simulink library "tqd"  (R2021b)
settings: Solver=VariableStepAuto  StartTime=0.0  StopTime=10.0  RelTol=1e-3
undefined symbols (not defined in the file or in its folder): ATQD_APSDecReq_X_kph, ATQD_APSDecReq_Y_mps2, ATQD_APSDecReqCMD_X_kph, ATQD_APSDecReqTs_X_pct, ATQD_APSDecTimeGain_X_Deg, ATQD_APSDecTimeGain_Y_s, ATQD_APSReqLowSpd_X_Deg, ATQD_AutoHoldReleaseBPS_X_Deg, ATQD_AWDLoadTrqnsGain_X_kg, ATQD_AWDLoadTrqnsGain_Y_pct, ATQD_BOSEnBPSPosn_X_kph, ATQD_BOSMap_X_rpm, ATQD_BOSMap_Y_pct, ATQD_CreepBaseTqD_X_kph, ATQD_CreepBaseTqD_Y_Deg, ATQD_CreepBaseTqR_X_kph, ATQD_CreepBaseTqR_Y_Deg, ATQD_CreepBPSDisPosn_X_Deg, ATQD_CreepBPSDisPosnR_X_Deg, ATQD_CreepBPSEnPosn_X_Deg, ATQD_CreepBPSEnPosnR_X_Deg, ATQD_CreepDeltaTq_X_kph, ATQD_CreepIterm_X_kph, ATQD_CreepIterm_Y_kph, ATQD_CreepItermMaxLimit_X_pct, ATQD_CreepPreloadTime_X_kph, ATQD_CreepPreloadTq_X_kph, ATQD_CreepPreloadTq_Y_s, ATQD_CreepProtTq_X_Deg, ATQD_CreepPterm_X_kph, ATQD_CreepPterm_Y_kph, ATQD_ECOTqMapD_X_rpm, ATQD_ECOTqMapD_Y_pct, ATQD_EOPDTqMapDCon_X_rpm, ATQD_EOPDTqMapDCon_Y_Deg, ATQD_EstInitVehWeight_X_c, ATQD_LHMRollGenMapD_X_rpm, ATQD_LHMRollGenMapD_Y_rpm, ATQD_LHMTqMapD_X_rpm, ATQD_LHMTqMapD_Y_pct, ATQD_NL1TqMapD_X_rpm, ATQD_NL1TqMapD_Y_pct, ATQD_NOPDTqMapDCon_X_rpm, ATQD_NOPDTqMapDCon_Y_Deg, ATQD_NRMRrEDUSpRat_X_rpm, ATQD_NRMRrEDUSpRat_Y_Nm, ATQD_OPDHoldDownRelDelay_X_Deg, ATQD_OPDHoldEnSpd_X_Deg, ATQD_OPDHoldRelDetTime_X_Deg, ATQD_OPDHoldReleaseTq_X_Deg, ATQD_OrigPedTqLowLim_X_Deg, ATQD_OrigPedTqLowLim_Y_pct, ATQD_PedalMapClimbUpLim_X_rpm, ATQD_PedalMapClimbUpLim_Y_Deg, ATQD_PreLoadTq_X_s, ATQD_RollGenMapEL1_X_rpm, ATQD_RollGenMapEL1_Y_rpm, ATQD_SL1TqMapD_X_rpm, ATQD_SL1TqMapD_Y_pct, ATQD_SlideRegenTqGain_X_Gps ... (+487)
libraries: hcu_lib x83, simulink x73, tqr x1
(part 14 of 19)

== system tqd/TQD/TorqueDemand/TorqueModule/AvaliableTqLimit/TorqueCapacityCalcalation/CapacityDistribution ==
  VTQD_FrEDUSpRat_cmd : Inport
  VTQD_RrEDUSpRat_rat : Inport  Port=2
  VTQD_TMPwrAvailDchrg_kW : Inport  Port=3
  VINP_HVBPwrAvailChrg_kw : Inport  Port=4
  Abs1 : Abs
  Product{,1,4..5} (4 alike) : Product
  VTQD_FrHVBPwrAvailDchrg_kw : Outport
  VTQD_RrHVBPwrAvailDchrg_kw : Outport  Port=2
  VTQD_FrHVBPwrAvailChrg_kw : Outport  Port=3
  VTQD_RrHVBPwrAvailChrg_kw : Outport  Port=4
  wires:
  VTQD_RrEDUSpRat_rat/1 -> [VTQD_RrEDUSpRat_rat]
  VTQD_FrEDUSpRat_cmd/1 -> [VTQD_FrEDUSpRat_rat]
  VINP_HVBPwrAvailChrg_kw/1 -> Abs1/1
  Product4/1 -> VTQD_FrHVBPwrAvailChrg_kw/1
  Product5/1 -> VTQD_RrHVBPwrAvailChrg_kw/1
  Product1/1 -> VTQD_RrHVBPwrAvailDchrg_kw/1  "VTQD_RrHVBPwrAvailDchrg_kW"
  [VTQD_FrEDUSpRat_rat] -> Product4/1
  [VTQD_FrEDUSpRat_rat] -> Product/1
  Abs1/1 -> Product4/2, Product5/1
  VTQD_TMPwrAvailDchrg_kW/1 -> Product1/1, Product/2
  [VTQD_RrEDUSpRat_rat] -> Product5/2
  Product/1 -> VTQD_FrHVBPwrAvailDchrg_kw/1  "VTQD_FrHVBPwrAvailDchrg_kW"
  [VTQD_RrEDUSpRat_rat] -> Product1/2

== system tqd/TQD/TorqueDemand/TorqueModule/AvaliableTqLimit/TorqueCapacityCalcalation/Generation ==
  VTQD_FrShaftSpd_rpm : Inport
  VTQD_RrShaftSpd_rpm : Inport  Port=2
  VTQD_FrHVBPwrAvailChrg_kw : Inport  Port=3
  VTQD_RrHVBPwrAvailChrg_kw : Inport  Port=4
  KTQD_FrBatapCont_factor : Inport  Port=5
  KTQD_RrBatapCont_factor : Inport  Port=6
  VINP_FrRegenAvailTq_Nm : Inport  Port=7
  VINP_RrRegenAvailTq_Nm : Inport  Port=8
  VTQD_GearActualPosn_enum : Inport  Port=9
  VINP_VehicleType_enum : Inport  Port=10
  Abs2 : Abs
  Abs6 : Abs
  Constant : Constant  Value=KTQD_WhlTqCapGenFr_Nm_ovrdflg
  Constant1 : Constant  Value=KTQD_WhlTqCapGenFr_Nm_ovrdval
  Constant10 : Constant  Value=ENUM_GEARACTUALPOSN_P  OutDataTypeStr=single
  Constant11 : Constant  Value=ENUM_GEARACTUALPOSN_P  OutDataTypeStr=single
  Constant12 : Constant  Value=ENUM_VEHICLETYPE_D31L24
  Constant13 : Constant  Value=ZERO_FLOAT
  Constant14 : Constant  Value=ENUM_GEARACTUALPOSN_N  OutDataTypeStr=single
  Constant19 : Constant  Value=ENUM_VEHICLETYPE_D31L24
  Constant2 : Constant  Value=KTQD_RrTMSpdMin_rpm  OutDataTypeStr=single
  Constant3 : Constant  Value=KTQD_WhlTqCapGenRr_Nm_ovrdflg
  Constant4 : Constant  Value=KTQD_RrTMTotalGearRatio_gain  OutDataTypeStr=single
  Constant5 : Constant  Value=KTQD_FrTMSpdMin_rpm  OutDataTypeStr=single
  Constant6 : Constant  Value=KTQD_FrTMTotalGearRatio_gain  OutDataTypeStr=single
  Constant7 : Constant  Value=KTQD_WhlTqCapGenRr_Nm_ovrdval
  Constant8 : Constant  Value=ZERO_FLOAT
  Constant9 : Constant  Value=ENUM_GEARACTUALPOSN_N  OutDataTypeStr=single
  Equal{1..4} (4 alike) : RelationalOperator  Operator===  OutDataTypeStr=boolean  RndMeth=Simplest
  Equal5 : RelationalOperator  Operator=~=  OutDataTypeStr=boolean  RndMeth=Simplest
  Equal6 : RelationalOperator  Operator=~=  OutDataTypeStr=boolean  RndMeth=Simplest
  Fcn : Fcn  Expr=u[1]/u[2]/pi*u[3]
  Fcn2 : Fcn  Expr=u[1]/u[2]/pi*u[3]
  Gain1 : Gain  Gain=-1
  Gain4 : Gain  Gain=-1
  Logical Operator1 : Logic  AllPortsSameDT=off  OutDataTypeStr=boolean
  Logical Operator2 : Logic  AllPortsSameDT=off  OutDataTypeStr=boolean
  Max{,1..2,4} (4 alike) : MinMax  Function=max  Inputs=2
  Mux : Mux  Inputs=3
  Mux2 : Mux  Inputs=3
  OR1 : Logic  Operator=OR  AllPortsSameDT=off  OutDataTypeStr=boolean
  OR2 : Logic  Operator=OR  AllPortsSameDT=off  OutDataTypeStr=boolean
  Product1 : Product
  Product2 : Product
  Saturation1 : Saturate  UpperLimit=0  LowerLimit=KTQD_FrLowTheldTrq_Nm
      settings: AttributesFormatString=|
      | Upper Limit :%<UpperLimit>
      | Lower Limit :%<LowerLimit>
  Saturation2 : Saturate  UpperLimit=0  LowerLimit=KTQD_RrLowTheldTrq_Nm
      settings: AttributesFormatString=|
      | Upper Limit :%<UpperLimit>
      | Lower Limit :%<LowerLimit>
  Switch : Switch  Criteria=u2 ~= 0
      settings: AttributesFormatString=<%<Criteria>>
  Switch1 : Switch  Criteria=u2 ~= 0
      settings: AttributesFormatString=<%<Criteria>>
  Switch2 : Switch  Criteria=u2 > Threshold
  Switch3 : Switch  Criteria=u2 > Threshold
  VTQD_WhlTqCapGenFr_Nm : Outport
  VTQD_WhlTqCapGenRr_Nm : Outport  Port=2
  wires:
  Gain1/1 -> Saturation2/1
  Gain4/1 -> Saturation1/1
  Switch1/1 -> VTQD_WhlTqCapGenRr_Nm/1  "VTQD_WhlTqCapGenRr_Nm"
  Constant3/1 -> Switch1/2
  Constant7/1 -> Switch1/1
  Switch/1 -> VTQD_WhlTqCapGenFr_Nm/1  "VTQD_WhlTqCapGenFr_Nm"
  Constant1/1 -> Switch/1
  Constant/1 -> Switch/2
  VTQD_RrHVBPwrAvailChrg_kw/1 -> [VTQD_RrHVBPwrAvailChrg_kw]
  KTQD_FrBatapCont_factor/1 -> [KTQD_FrBatapCont_factor]
  VTQD_FrHVBPwrAvailChrg_kw/1 -> [VTQD_FrHVBPwrAvailChrg_kw]
  VTQD_FrShaftSpd_rpm/1 -> [VTQD_FrShaftSpd_rpm]
  VTQD_RrShaftSpd_rpm/1 -> [VTQD_RrShaftSpd_rpm]
  KTQD_RrBatapCont_factor/1 -> [KTQD_RrBatapCont_factor]
  Fcn2/1 -> Gain1/1
  Max1/1 -> Mux2/2
  Abs2/1 -> Max1/1
  Mux2/1 -> Fcn2/1
  Constant2/1 -> Max1/2
  [KTQD_RrBatapCont_factor] -> Mux2/3
  [VTQD_RrShaftSpd_rpm] -> Abs2/1
  [VTQD_RrHVBPwrAvailChrg_kw] -> Mux2/1
  Fcn/1 -> Gain4/1
  Abs6/1 -> Max4/1
  [VTQD_FrHVBPwrAvailChrg_kw] -> Mux/1
  Constant5/1 -> Max4/2
  [VTQD_FrShaftSpd_rpm] -> Abs6/1
  [KTQD_FrBatapCont_factor] -> Mux/3
  Mux/1 -> Fcn/1
  Max4/1 -> Mux/2
  Saturation1/1 -> Max2/1
  Max2/1 -> Switch/3
  Saturation2/1 -> Max/1
  Max/1 -> Switch1/3
  VINP_RrRegenAvailTq_Nm/1 -> [VINP_RrRegenAvailTq_Nm]
  VINP_FrRegenAvailTq_Nm/1 -> [VINP_FrRegenAvailTq_Nm]
  VTQD_GearActualPosn_enum/1 -> [VTQD_GearActualPosn_enum]
  [VINP_FrRegenAvailTq_Nm] -> Product2/1
  Equal2/1 -> OR2/2
  Equal4/1 -> OR2/1
  Constant10/1 -> Equal4/2
  Constant6/1 -> Product2/2
  Constant9/1 -> Equal2/2
  [VTQD_GearActualPosn_enum] -> Equal2/1
  Constant8/1 -> Switch2/1
  Product2/1 -> Switch2/3
  [VTQD_GearActualPosn_enum] -> Equal4/1
  Switch2/1 -> Max2/2
  Constant4/1 -> Product1/2
  [VINP_RrRegenAvailTq_Nm] -> Product1/1
  Switch3/1 -> Max/2
  [VINP_VehicleType_enum] -> Equal6/1
  Equal6/1 -> Logical Operator1/2
  Constant19/1 -> Equal6/2
  OR2/1 -> Logical Operator1/1
  Logical Operator1/1 -> Switch2/2
  OR1/1 -> Logical Operator2/1
  Equal5/1 -> Logical Operator2/2
  Constant12/1 -> Equal5/2
  [VINP_VehicleType_enum] -> Equal5/1
  Constant14/1 -> Equal1/2
  Equal1/1 -> OR1/2
  Constant13/1 -> Switch3/1
  [VTQD_GearActualPosn_enum] -> Equal1/1
  Constant11/1 -> Equal3/2
  [VTQD_GearActualPosn_enum] -> Equal3/1
  Logical Operator2/1 -> Switch3/2
  Equal3/1 -> OR1/1
  Product1/1 -> Switch3/3
  VINP_VehicleType_enum/1 -> [VINP_VehicleType_enum]

== system tqd/TQD/TorqueDemand/TorqueModule/AvaliableTqLimit/TorqueCapacityCalcalation/Motoring ==
  VTQD_FrShaftSpd_rpm : Inport
  VTQD_RrShaftSpd_rpm : Inport  Port=2
  VTQD_FrHVBPwrAvailDchrg_kw : Inport  Port=3
  VTQD_RrHVBPwrAvailDchrg_kw : Inport  Port=4
  KTQD_FrBatapCont_factor : Inport  Port=5
  KTQD_RrBatapCont_factor : Inport  Port=6
  VINP_HVBCellVoltMax_mV : Inport  Port=7
  VINP_HVBCellVoltMin_mV : Inport  Port=8
  VINP_HVBSOH_pct : Inport  Port=9
  VINP_FrMotorAvailTq_Nm : Inport  Port=10
  VINP_RrMotorAvailTq_Nm : Inport  Port=11
  VTQD_GearActualPosn_enum : Inport  Port=12
  VINP_VehicleType_enum : Inport  Port=13
  Abs : Abs
  Abs2 : Abs
  Add : Sum  Commented=on  Inputs=+-
  Constant : Constant  Value=KTQD_WhlTqCapMotFr_Nm_ovrdflg
  Constant1 : Constant  Value=KTQD_FrTMSpdMin_rpm  OutDataTypeStr=single
  Constant10 : Constant  Value=KTQD_FrTMTotalGearRatio_gain  OutDataTypeStr=single
  Constant11 : Constant  Value=KTQD_RrTMTotalGearRatio_gain  OutDataTypeStr=single
  Constant{2,4,12..13} (4 alike) : Constant  Value=ZERO_FLOAT
  Constant14 : Constant  Value=ENUM_GEARACTUALPOSN_N  OutDataTypeStr=single
  Constant15 : Constant  Value=ENUM_GEARACTUALPOSN_P  OutDataTypeStr=single
  Constant16 : Constant  Value=ENUM_GEARACTUALPOSN_N  OutDataTypeStr=single
  Constant17 : Constant  Value=ENUM_GEARACTUALPOSN_P  OutDataTypeStr=single
  Constant18 : Constant  Value=ENUM_VEHICLETYPE_D31L24
  Constant19 : Constant  Value=ENUM_VEHICLETYPE_D31L24
  Constant3 : Constant  Value=KTQD_RrTMSpdMin_rpm  OutDataTypeStr=single
  Constant5 : Constant  Value=KTQD_WhlTqCapMotFr_Nm_ovrdval
  Constant6 : Constant  Value=KTQD_WhlTqCapMotRr_Nm_ovrdflg
  Constant7 : Constant  Value=KTQD_WhlTqCapMotRr_Nm_ovrdval
  Constant8 : Constant  Value=KTQD_FrUppTheldTrq_Nm
  Constant9 : Constant  Value=KTQD_RrUppTheldTrq_Nm
  Equal{1..3,5} (4 alike) : RelationalOperator  Operator===  OutDataTypeStr=boolean  RndMeth=Simplest
  Equal4 : RelationalOperator  Operator=~=  OutDataTypeStr=boolean  RndMeth=Simplest
  Equal6 : RelationalOperator  Operator=~=  OutDataTypeStr=boolean  RndMeth=Simplest
  Fcn : Fcn  Expr=u[1]/u[2]/pi*u[3]
  Fcn2 : Fcn  Expr=u[1]/u[2]/pi*u[3]
  From3 : From  Commented=on  GotoTag=VINP_HVBCellVoltMax_mV
  From4 : From  Commented=on  GotoTag=VINP_HVBCellVoltMin_mV
  From5 : From  Commented=on  GotoTag=VTQD_HCBCellVoltDev_mV
  From6 : From  Commented=on  GotoTag=VINP_HVBSOH_pct
  Goto7 : Goto  Commented=on  GotoTag=VTQD_HCBCellVoltDev_mV
  Goto9 : Goto  Commented=on  GotoTag=VTQD_WhlTqCapMotGain_c
  Logical Operator : Logic  AllPortsSameDT=off  OutDataTypeStr=boolean
  Logical Operator1 : Logic  AllPortsSameDT=off  OutDataTypeStr=boolean
  MTQD_WhlTqCapMotGain_Z_c : Lookup_n-D  Commented=on  BreakpointsForDimension1=ATQD_WhlTqCapMotGain_Y_mV  BreakpointsForDimension2=ATQD_WhlTqCapMotGain_X_pct  Table=MTQD_WhlTqCapMotGain_Z_c  InternalRulePriority=Speed  RndMeth=Simplest  InputSameDT=on
      settings: InputPortMap=u0,u1
  Max{,1..3} (4 alike) : MinMax  Function=max  Inputs=2
  Min : MinMax  Inputs=3
  Min1 : MinMax  Inputs=3
  Mux : Mux  Inputs=3
  Mux2 : Mux  Inputs=3
  OR1 : Logic  Operator=OR  AllPortsSameDT=off  OutDataTypeStr=boolean
  OR2 : Logic  Operator=OR  AllPortsSameDT=off  OutDataTypeStr=boolean
  Product : Product
  Product1 : Product
  Switch : Switch  Criteria=u2 ~= 0
      settings: AttributesFormatString=<%<Criteria>>
  Switch1 : Switch  Criteria=u2 ~= 0
      settings: AttributesFormatString=<%<Criteria>>
  Switch2 : Switch  Criteria=u2 > Threshold
  Switch3 : Switch  Criteria=u2 > Threshold
  VTQD_WhlTqCapMotFr_Nm : Outport
  VTQD_WhlTqCapMotRr_Nm : Outport  Port=2
  wires:
  Fcn2/1 -> Min1/1
  Switch1/1 -> VTQD_WhlTqCapMotRr_Nm/1  "VTQD_WhlTqCapMotRr_Nm"
  Constant7/1 -> Switch1/1
  Constant6/1 -> Switch1/2
  Constant5/1 -> Switch/1
  Constant/1 -> Switch/2
  Switch/1 -> VTQD_WhlTqCapMotFr_Nm/1  "VTQD_WhlTqCapMotFr_Nm"
  VTQD_RrHVBPwrAvailDchrg_kw/1 -> [VTQD_RrHVBPwrAvailDchrg_kw]
  KTQD_RrBatapCont_factor/1 -> [KTQD_RrBatapCont_factor]
  VTQD_RrShaftSpd_rpm/1 -> [VTQD_RrShaftSpd_rpm]
  Abs2/1 -> Max2/1
  [VTQD_RrHVBPwrAvailDchrg_kw] -> Mux2/1
  Constant3/1 -> Max2/2
  [VTQD_RrShaftSpd_rpm] -> Abs2/1
  Mux2/1 -> Fcn2/1
  Max2/1 -> Mux2/2
  [VTQD_FrHVBPwrAvailDchrg_kw] -> Mux/1
  Max/1 -> Mux/2
  [VTQD_FrShaftSpd_rpm] -> Abs/1
  KTQD_FrBatapCont_factor/1 -> [KTQD_FrBatapCont_factor]
  VTQD_FrHVBPwrAvailDchrg_kw/1 -> [VTQD_FrHVBPwrAvailDchrg_kw]
  Abs/1 -> Max/1
  Fcn/1 -> Min/1
  Mux/1 -> Fcn/1
  VTQD_FrShaftSpd_rpm/1 -> [VTQD_FrShaftSpd_rpm]
  Constant1/1 -> Max/2
  Constant8/1 -> Min/2
  Min/1 -> Max1/1
  Constant2/1 -> Max1/2
  Constant9/1 -> Min1/2
  Constant4/1 -> Max3/2
  VINP_HVBCellVoltMin_mV/1 -> [VINP_HVBCellVoltMin_mV]
  VINP_HVBSOH_pct/1 -> [VINP_HVBSOH_pct]
  VINP_HVBCellVoltMax_mV/1 -> [VINP_HVBCellVoltMax_mV]
  Add/1 -> Goto7/1  "VTQD_HCBCellVoltDev_mV"
  From3/1 -> Add/1
  From4/1 -> Add/2
  From5/1 -> MTQD_WhlTqCapMotGain_Z_c/1
  [KTQD_FrBatapCont_factor] -> Mux/3
  [KTQD_RrBatapCont_factor] -> Mux2/3
  MTQD_WhlTqCapMotGain_Z_c/1 -> Goto9/1  "VTQD_WhlTqCapMotGain_c"
  Max1/1 -> Switch/3
  Max3/1 -> Switch1/3
  From6/1 -> MTQD_WhlTqCapMotGain_Z_c/2
  VINP_FrMotorAvailTq_Nm/1 -> [VINP_FrMotorAvailTq_Nm]
  VINP_RrMotorAvailTq_Nm/1 -> [VINP_RrMotorAvailTq_Nm]
  Min1/1 -> Max3/1
  Constant10/1 -> Product/2
  [VINP_FrMotorAvailTq_Nm] -> Product/1
  Constant16/1 -> Equal1/2
  Constant11/1 -> Product1/2
  Switch3/1 -> Min1/3
  [VINP_RrMotorAvailTq_Nm] -> Product1/1
  Equal3/1 -> OR1/1
  [VTQD_GearActualPosn_enum] -> Equal3/1
  Product1/1 -> Switch3/3
  Constant13/1 -> Switch3/1
  [VTQD_GearActualPosn_enum] -> Equal1/1
  Equal1/1 -> OR1/2
  Constant17/1 -> Equal3/2
  VTQD_GearActualPosn_enum/1 -> [VTQD_GearActualPosn_enum]
  [VINP_VehicleType_enum] -> Equal4/1
  Equal4/1 -> Logical Operator/2
  Constant18/1 -> Equal4/2
  OR1/1 -> Logical Operator/1
  Logical Operator/1 -> Switch3/2
  Equal6/1 -> Logical Operator1/2
  [VINP_VehicleType_enum] -> Equal6/1
  Constant19/1 -> Equal6/2
  Constant14/1 -> Equal2/2
  Equal5/1 -> OR2/1
  [VTQD_GearActualPosn_enum] -> Equal5/1
  Equal2/1 -> OR2/2
  Constant15/1 -> Equal5/2
  Constant12/1 -> Switch2/1
  Switch2/1 -> Min/3
  OR2/1 -> Logical Operator1/1
  Logical Operator1/1 -> Switch2/2
  [VTQD_GearActualPosn_enum] -> Equal2/1
  Product/1 -> Switch2/3
  VINP_VehicleType_enum/1 -> [VINP_VehicleType_enum]

== system tqd/TQD/TorqueDemand/TorqueModule/AvaliableTqLimit/TorqueCapacityCalcalation/TMAvailablePwr_Calculation ==
  VINP_HVBPwrAvailDchrg_kw : Inport
  Add : Sum
  Constant : Constant  Value=KTQD_DCDCCalPwrAvailRsv_kW
  Constant1 : Constant  Value=KTQD_THCMCalPwrAvailRsv_kW
  Constant2 : Constant  Value=KTQD_TMPwrAvailDchrg_kW_ovrdflg
  Constant3 : Constant  Value=ZERO_FLOAT
  Min : MinMax  Function=max  Inputs=2
  Subtract : Sum  Inputs=+-
  Switch : Switch  Criteria=u2 ~= 0
      settings: AttributesFormatString=<%<Criteria>>
  VTQD_TMPwrAvailDchrg_kW : Outport
  wires:
  Constant3/1 -> Min/2
  Min/1 -> Switch/1
  Switch/1 -> VTQD_TMPwrAvailDchrg_kW/1  "VTQD_TMPwrAvailDchrg_kW"
  Constant2/1 -> Switch/2
  Subtract/1 -> Min/1
  Add/1 -> Subtract/2
  VINP_HVBPwrAvailDchrg_kw/1 -> Subtract/1, Switch/3
  Constant1/1 -> Add/2
  Constant/1 -> Add/1

== system tqd/TQD/TorqueDemand/TorqueModule/DriverWhlTqDem/Creep/If Action Subsystem ==
  In1 : Inport
  Action Port : ActionPort
  Out1 : Outport
  wires:
  In1/1 -> Out1/1

== system tqd/TQD/TorqueDemand/TorqueModule/DriverWhlTqDem/Creep/If Action Subsystem1 ==
  VTQD_ActBPSPosnInRange_flg : Inport
  VTQD_CreepErrSpd_kph : Inport  Port=2
  VTQD_CreepPterm_c : Inport  Port=3
  VTQD_CreepIterm_c : Inport  Port=4
  VTQD_CreepDeltaTq_Nm : Inport  Port=5
  VTQD_ActBPSPosn_pct : Inport  Port=6
  task_time_s : Inport  Port=7
  VTQD_CreepDisable_flg : Inport  Port=8
  VTQD_CreepEnable_flg : Inport  Port=9
  VTQD_OPDOn2Off : Inport  Port=10
  Add : Sum
  Add1 : Sum  Inputs=+++
  Constant : Constant  Value=ZERO_FLOAT
  Constant1 : Constant  Value=KTQD_CreepItermMinLimit_Nm
  Constant4 : Constant  Value=ZERO_FLOAT
  Constant5 : Constant  Value=ONE_FLOAT
  Data Type Conversion : DataTypeConversion
  Goto1 : Goto  Commented=on  GotoTag=VTQD_CreepErrSpd_kph
  Goto10 : Goto  Commented=on  GotoTag=VTQD_CreepTotalOfstTq_Nm
  Goto6 : Goto  Commented=on  GotoTag=task_time_s
  Goto7 : Goto  Commented=on  GotoTag=VTQD_CreepPtermTq_Nm
  Goto8 : Goto  Commented=on  GotoTag=VTQD_CreepItermTq_Nm
  Goto9 : Goto  Commented=on  GotoTag=VTQD_CreepOffsetTq_Nm
  Ground{1..6} (6 alike) : Ground  Commented=on
  MTQD_CreepItermMaxLimit_Y_Nm : Lookup_n-D  NumberOfTableDimensions=1  BreakpointsForDimension1=ATQD_CreepItermMaxLimit_X_pct  Table=MTQD_CreepItermMaxLimit_Y_Nm  ExtrapMethod=Clip  InternalRulePriority=Speed  RndMeth=Simplest  InputSameDT=on
  NOT : Logic  Operator=NOT  AllPortsSameDT=off  OutDataTypeStr=boolean
  OR : Logic  Operator=OR  Inputs=4  AllPortsSameDT=off  OutDataTypeStr=boolean
  Product : Product
  Product2 : Product
  Saturation Dynamic : simulink/Discontinuities/Saturation Dynamic  OutMin=[]  OutMax=[]  OutDataTypeStr=Inherit: Same as second input  OutDataType=fixdt(1, 16)  OutScaling=2^-10  DoSatur=off
  Switch1 : Switch  Criteria=u2 ~= 0
  Switch4 : Switch  Criteria=u2 ~= 0
  Terminator1 : Terminator
  Terminator2 : Terminator
  Unit Delay : UnitDelay  SampleTime=-1  HasFrameUpgradeWarning=on
  VTQD_CreepTotalOfstTq_Nm : Outport
  wires:
  Add1/1 -> VTQD_CreepTotalOfstTq_Nm/1  "VTQD_CreepTotalOfstTq_Nm"
  VTQD_CreepDeltaTq_Nm/1 -> [VTQD_CreepDeltaTq_Nm]
  VTQD_CreepIterm_c/1 -> [VTQD_CreepIterm_c]
  VTQD_CreepPterm_c/1 -> [VTQD_CreepPterm_c]
  VTQD_ActBPSPosnInRange_flg/1 -> [VTQD_ActBPSPosnInRange_flg]
  task_time_s/1 -> Terminator1/1
  VTQD_ActBPSPosn_pct/1 -> [VTQD_ActBPSPosn_pct]
  Ground1/1 -> Goto6/1
  Ground2/1 -> Goto7/1
  Ground3/1 -> Goto8/1
  Ground4/1 -> Goto9/1
  Ground5/1 -> Goto10/1
  VTQD_CreepErrSpd_kph/1 -> Terminator2/1
  Ground6/1 -> Goto1/1
  VTQD_CreepDisable_flg/1 -> [VTQD_CreepDisable_flg]
  OR/1 -> [VTQD_CreepPICtrlReset_flg]  "VTQD_CreepPICtrlReset_flg"
  VTQD_CreepEnable_flg/1 -> [VTQD_CreepEnable_flg]
  VTQD_OPDOn2Off/1 -> [VTQD_OPDOn2Off_flg]
  [VTQD_OPDOn2Off_flg] -> OR/2
  [VTQD_CreepDisable_flg] -> OR/3
  [VTQD_ActBPSPosnInRange_flg] -> OR/1
  [VTQD_CreepEnable_flg] -> NOT/1
  NOT/1 -> OR/4
  Data Type Conversion/1 -> Add1/3  "VTQD_CreepOffsetTq_Nm"
  Constant1/1 -> Saturation Dynamic/3
  [VTQD_ActBPSPosn_pct] -> MTQD_CreepItermMaxLimit_Y_Nm/1
  [VTQD_CreepPICtrlReset_flg] -> Switch4/2
  MTQD_CreepItermMaxLimit_Y_Nm/1 -> Saturation Dynamic/1  "VTQD_CreepItermMaxLimit_Nm"
  Constant/1 -> Switch1/1
  Product/1 -> Switch1/3
  [VTQD_CreepPterm_c] -> Product/1
  Constant5/1 -> Product/2, Product2/1
  [VTQD_CreepPICtrlReset_flg] -> Switch1/2
  Add/1 -> Switch4/3
  Switch1/1 -> Add1/1  "VTQD_CreepPtermTq_Nm"
  Saturation Dynamic/1 -> Add1/2  "VTQD_CreepItermTq_Nm"
  Product2/1 -> Add/1
  Switch4/1 -> Unit Delay/1, Saturation Dynamic/2
  Unit Delay/1 -> Add/2
  Constant4/1 -> Switch4/1
  [VTQD_CreepIterm_c] -> Product2/2
  [VTQD_CreepDeltaTq_Nm] -> Data Type Conversion/1

== system tqd/TQD/TorqueDemand/TorqueModule/DriverWhlTqDem/Creep/Switch Case Action Subsystem ==
  In1 : Inport
  Action Port : ActionPort
  Out1 : Outport
  wires:
  In1/1 -> Out1/1

== system tqd/TQD/TorqueDemand/TorqueModule/DriverWhlTqDem/PedalMapWhlTq/LHM ==
  VTQD_ActAPSPosn_pct : Inport
  VTQD_TqTargetShaftSpd_rpm : Inport  Port=2
  VTQD_RollRegenEnable_flg : Inport  Port=3
  VTQD_RollingShaftSpd_rpm : Inport  Port=4
  VTQD_GearActualPosn_enum : Inport  Port=5
  Action Port : ActionPort
  Constant : Constant  Value=ZERO_FLOAT
  Constant1 : Constant  Value=ENUM_GEARACTUALPOSN_D
  Constant11 : Constant  Commented=on  Value=ENUM_GEARACTUALPOSN_D
  Constant12 : Constant  Commented=on  Value=ENUM_GEARACTUALPOSN_R
  Constant2 : Constant  Value=ENUM_GEARACTUALPOSN_R
  Equal1 : RelationalOperator  Operator===  OutDataTypeStr=boolean  RndMeth=Simplest
  Equal2 : RelationalOperator  Operator===  OutDataTypeStr=boolean  RndMeth=Simplest
  Equal7 : RelationalOperator  Commented=on  Operator===  OutDataTypeStr=boolean  RndMeth=Simplest
  Equal8 : RelationalOperator  Commented=on  Operator===  OutDataTypeStr=boolean  RndMeth=Simplest
  From22 : From  Commented=on  GotoTag=VTQD_GearActualPosn_enum
  From23 : From  Commented=on  GotoTag=VTQD_GearActualPosn_enum
  From24 : From  Commented=on  GotoTag=VTQD_ActAPSPosn_pct
  From25 : From  Commented=on  GotoTag=VTQD_TqTargetShaftSpd_rpm
  From39 : From  Commented=on  GotoTag=VTQD_ActAPSPosn_pct
  From40 : From  Commented=on  GotoTag=VTQD_TqTargetShaftSpd_rpm
  From8 : From  Commented=on  GotoTag=VTQD_RollRegenEnable_flg
  From9 : From  Commented=on  GotoTag=VTQD_RollingShaftSpd_rpm
  GearShiftCheck : If  Commented=on  NumInputs=2  IfExpression=u1~= 0  ElseIfExpressions=u2~= 0
  MTQD_LHMTqMapD_Z_Nm : Lookup_n-D  BreakpointsForDimension1=ATQD_NL1TqMapD_Y_pct  BreakpointsForDimension2=ATQD_NL1TqMapD_X_rpm  Table=MTQD_LHMTqMapD_Z_Nm  ExtrapMethod=Clip  InternalRulePriority=Speed  RndMeth=Simplest  InputSameDT=on
      settings: InputPortMap=u0,u1
  MTQD_LHMTqMapR_Z_Nm : Lookup_n-D  BreakpointsForDimension1=ATQD_NL1TqMapD_Y_pct  BreakpointsForDimension2=ATQD_NL1TqMapD_X_rpm  Table=MTQD_LHMTqMapR_Z_Nm  ExtrapMethod=Clip  InternalRulePriority=Speed  RndMeth=Simplest  InputSameDT=on
      settings: InputPortMap=u0,u1
  Merge1 : Merge  Commented=on  Inputs=3
  ShiftD : Subsystem  Commented=on  TreatAsAtomicUnit=on
  ShiftPorN : Subsystem  Commented=on  TreatAsAtomicUnit=on
  ShiftR : Subsystem  Commented=on  TreatAsAtomicUnit=on
  Switch1 : Switch  Criteria=u2 ~= 0
  Switch2 : Switch  Criteria=u2 ~= 0
  Terminator : Terminator
  VTQD_PedalMapWhlTqLHM_Nm : Outport
  wires:
  Switch1/1 -> VTQD_PedalMapWhlTqLHM_Nm/1
  Constant/1 -> Switch2/3
  [VTQD_LHMTqMapR_Nm] -> Switch2/1
  Equal2/1 -> Switch2/2
  Constant2/1 -> Equal2/2
  [VTQD_GearActualPosn_enum] -> Equal2/1
  Switch2/1 -> Switch1/3
  [VTQD_LHMTqMapD_Nm] -> Switch1/1
  Constant1/1 -> Equal1/2
  Equal1/1 -> Switch1/2
  [VTQD_GearActualPosn_enum] -> Equal1/1
  [VTQD_TqTargetShaftSpd_rpm] -> MTQD_LHMTqMapR_Z_Nm/2
  [VTQD_ActAPSPosn_pct] -> MTQD_LHMTqMapR_Z_Nm/1
  MTQD_LHMTqMapR_Z_Nm/1 -> [VTQD_LHMTqMapR_Nm]
  MTQD_LHMTqMapD_Z_Nm/1 -> [VTQD_LHMTqMapD_Nm]
  [VTQD_TqTargetShaftSpd_rpm] -> MTQD_LHMTqMapD_Z_Nm/2
  [VTQD_ActAPSPosn_pct] -> MTQD_LHMTqMapD_Z_Nm/1
  VTQD_GearActualPosn_enum/1 -> [VTQD_GearActualPosn_enum]
  VTQD_RollingShaftSpd_rpm/1 -> [VTQD_RollingShaftSpd_rpm]
  VTQD_RollRegenEnable_flg/1 -> Terminator/1
  VTQD_TqTargetShaftSpd_rpm/1 -> [VTQD_TqTargetShaftSpd_rpm]
  VTQD_ActAPSPosn_pct/1 -> [VTQD_ActAPSPosn_pct]
  From25/1 -> ShiftR/2(VTQD_TqTargetShaftSpd_rpm)
  Constant12/1 -> Equal8/2
  From9/1 -> ShiftD/4(VTQD_RollingShaftSpd_rpm)
  GearShiftCheck/1 -> ShiftD/Action
  GearShiftCheck/3 -> ShiftPorN/Action
  Equal7/1 -> GearShiftCheck/1
  Constant11/1 -> Equal7/2
  ShiftD/1(VTQD_PedalMapWhlTqLHMD_Nm) -> Merge1/1
  From23/1 -> Equal8/1
  From39/1 -> ShiftD/1(VTQD_ActAPSPosn_pct)
  From22/1 -> Equal7/1
  GearShiftCheck/2 -> ShiftR/Action
  From8/1 -> ShiftD/3(VTQD_RollRegenEnable_flg)
  From40/1 -> ShiftD/2(VTQD_TqTargetShaftSpd_rpm)
  ShiftPorN/1(VTQD_PedalMapWhlTqPorN_Nm) -> Merge1/3
  From24/1 -> ShiftR/1(VTQD_ActAPSPosn_pct)
  Equal8/1 -> GearShiftCheck/2
  ShiftR/1(VTQD_PedalMapWhlTqLHMR_Nm) -> Merge1/2

== system tqd/TQD/TorqueDemand/TorqueModule/DriverWhlTqDem/PedalMapWhlTq/NoLHM ==
  VTQD_ActAPSPosn_pct : Inport
  VTQD_TqTargetShaftSpd_rpm : Inport  Port=2
  VTQD_RegenMode_enum : Inport  Port=3
  VTQD_RollRegenEnable_flg : Inport  Port=4
  VTQD_RollingShaftSpd_rpm : Inport  Port=5
  VTQD_GearActualPosn_enum : Inport  Port=6
  VTQD_EVDriveMode_enum : Inport  Port=7
  VVMC_EstSlope_Deg : Inport  Port=8
  VTQD_APSReqTimer_s : Inport  Port=9
  VTQD_LowIdleAccPedal_flg : Inport  Port=10
  VTQD_OPDHoldEnRel_flg : Inport  Port=11
  VTQD_OPDHoldActRelTq_Nm : Inport  Port=12
  VTQD_VehActSpd_kph : Inport  Port=13
  VTQD_SlopeUp_flg : Inport  Port=14
  VINP_IVISnowModeCmd_flg : Inport  Port=15
  VTQD_PreDecTqLowLim_Nm : Inport  Port=16
  Action Port : ActionPort  ActionPortLabel=else
  Constant11 : Constant  Value=ENUM_GEARACTUALPOSN_D
  Constant12 : Constant  Value=ENUM_GEARACTUALPOSN_R
  Equal7 : RelationalOperator  Operator===  OutDataTypeStr=boolean  RndMeth=Simplest
  Equal8 : RelationalOperator  Operator===  OutDataTypeStr=boolean  RndMeth=Simplest
  GearShiftCheck : If  NumInputs=2  IfExpression=u1~= 0  ElseIfExpressions=u2~= 0
  Merge1 : Merge  Inputs=3
  ShiftD : Subsystem  TreatAsAtomicUnit=on
  ShiftPorN : Subsystem  TreatAsAtomicUnit=on
  ShiftR : Subsystem  TreatAsAtomicUnit=on
  VTQD_PedalMapWhlTqNoLHM_Nm : Outport
  wires:
  [VTQD_RollingShaftSpd_rpm] -> ShiftD/6(VTQD_RollingShaftSpd_rpm)
  [VTQD_RollRegenEnable_flg] -> ShiftD/5(VTQD_RollRegenEnable_flg)
  ShiftR/1(VTQD_PedalMapWhlTqR_Nm) -> Merge1/2
  VTQD_EVDriveMode_enum/1 -> [VTQD_EVDriveMode_enum]
  VTQD_GearActualPosn_enum/1 -> [VTQD_GearActualPosn_enum]
  [VTQD_TqTargetShaftSpd_rpm] -> ShiftD/3(VTQD_TqTargetShaftSpd_rpm)
  Equal7/1 -> GearShiftCheck/1
  GearShiftCheck/3 -> ShiftPorN/Action
  Equal8/1 -> GearShiftCheck/2
  [VTQD_ActAPSPosn_pct] -> ShiftR/1(VTQD_ActAPSPosn_pct)
  ShiftPorN/1(VTQD_PedalMapWhlTqPorN_Nm) -> Merge1/3
  [VTQD_EVDriveMode_enum] -> ShiftD/1(VTQD_EVDriveMode_enum)
  [VTQD_TqTargetShaftSpd_rpm] -> ShiftR/2(VTQD_TqTargetShaftSpd_rpm)
  GearShiftCheck/1 -> ShiftD/Action
  Merge1/1 -> VTQD_PedalMapWhlTqNoLHM_Nm/1  "VTQD_PedalMapWhlTqNoLHM_Nm"
  Constant12/1 -> Equal8/2
  Constant11/1 -> Equal7/2
  GearShiftCheck/2 -> ShiftR/Action
  [VTQD_GearActualPosn_enum] -> Equal7/1
  [VTQD_ActAPSPosn_pct] -> ShiftD/2(VTQD_ActAPSPosn_pct)
  [VTQD_GearActualPosn_enum] -> Equal8/1
  ShiftD/1(VTQD_PedalMapWhlTqD_Nm) -> Merge1/1
  VTQD_RollingShaftSpd_rpm/1 -> [VTQD_RollingShaftSpd_rpm]
  VTQD_RollRegenEnable_flg/1 -> [VTQD_RollRegenEnable_flg]
  VTQD_RegenMode_enum/1 -> [VTQD_RegenMode_enum]
  VTQD_ActAPSPosn_pct/1 -> [VTQD_ActAPSPosn_pct]
  VTQD_TqTargetShaftSpd_rpm/1 -> [VTQD_TqTargetShaftSpd_rpm]
  [VVMC_EstSlope_Deg] -> ShiftD/7(VVMC_EstSlope_Deg)
  [VTQD_APSReqTimer_s] -> ShiftD/8(VTQD_APSReqTimer_s)
  VVMC_EstSlope_Deg/1 -> [VVMC_EstSlope_Deg]
  VTQD_APSReqTimer_s/1 -> [VTQD_APSReqTimer_s]
  [VTQD_RegenMode_enum] -> ShiftD/4(VTQD_RegenMode_enum)
  [VTQD_LowIdleAccPedal_flg] -> ShiftD/9(VTQD_LowIdleAccPedal_flg)
  VTQD_LowIdleAccPedal_flg/1 -> [VTQD_LowIdleAccPedal_flg]
  VTQD_OPDHoldEnRel_flg/1 -> [VTQD_OPDHoldEnRel_flg]
  [VTQD_OPDHoldEnRel_flg] -> ShiftD/10(VTQD_OPDHoldEnRel_flg)
  VTQD_OPDHoldActRelTq_Nm/1 -> [VTQD_OPDHoldActRelTq_Nm]
  VTQD_VehActSpd_kph/1 -> [VTQD_VehActSpd_kph]
  [VTQD_OPDHoldActRelTq_Nm] -> ShiftD/11(VTQD_OPDHoldActRelTq_Nm)
  [VTQD_VehActSpd_kph] -> ShiftD/12(VTQD_VehActSpd_kph)
  VTQD_SlopeUp_flg/1 -> [VTQD_SlopeUp_flg]
  [VTQD_SlopeUp_flg] -> ShiftD/13(VTQD_SlopeUp_flg)
  [VINP_IVISnowModeCmd_flg] -> ShiftD/14(VINP_IVISnowModeCmd_flg)
  [VTQD_PreDecTqLowLim_Nm] -> ShiftD/15(VTQD_PreDecTqLowLim_Nm)
  VTQD_PreDecTqLowLim_Nm/1 -> [VTQD_PreDecTqLowLim_Nm]
  VINP_IVISnowModeCmd_flg/1 -> [VINP_IVISnowModeCmd_flg]

== system tqd/TQD/TorqueDemand/TorqueModule/DriverWhlTqDem/PedalMapWhlTq/Triggered Subsystem ==
  in1 : Inport
  In2 : Inport  Port=2
  Trigger : TriggerPort  VariantControl=(inherit)
  Out1 : Outport
  Out2 : Outport  Port=2
  wires:
  in1/1 -> Out1/1
  In2/1 -> Out2/1

== system tqd/TQD/TorqueDemand/TorqueModule/DriverWhlTqDem/PedalMapWhlTq/LHM/ShiftD ==
  VTQD_ActAPSPosn_pct : Inport
  VTQD_TqTargetShaftSpd_rpm : Inport  Port=2
  VTQD_RollRegenEnable_flg : Inport  Port=3
  VTQD_RollingShaftSpd_rpm : Inport  Port=4
  Action Port : ActionPort
  MTQD_LHMRollGenMapD_Z_Nm : Lookup_n-D  BreakpointsForDimension1=ATQD_LHMRollGenMapD_Y_rpm  BreakpointsForDimension2=ATQD_LHMRollGenMapD_X_rpm  Table=MTQD_LHMRollGenMapD_Z_Nm  InternalRulePriority=Speed  RndMeth=Simplest  InputSameDT=on
      settings: InputPortMap=u0,u1
  MTQD_LHMTqMapD_Z_Nm : Lookup_n-D  BreakpointsForDimension1=ATQD_LHMTqMapD_Y_pct  BreakpointsForDimension2=ATQD_LHMTqMapD_X_rpm  Table=MTQD_LHMTqMapD_Z_Nm  InternalRulePriority=Speed  RndMeth=Simplest  InputSameDT=on
      settings: InputPortMap=u0,u1
  Switch : Switch  Criteria=u2 ~= 0
  VTQD_PedalMapWhlTqLHMD_Nm : Outport
  wires:
  Switch/1 -> VTQD_PedalMapWhlTqLHMD_Nm/1
  [MTQD_LHMTqMapD_Z_Nm] -> Switch/3
  [MTQD_LHMRollGenMapD_Z_Nm] -> Switch/1
  [VTQD_RollRegenEnable_flg] -> Switch/2
  MTQD_LHMRollGenMapD_Z_Nm/1 -> [MTQD_LHMRollGenMapD_Z_Nm]
  [VTQD_TqTargetShaftSpd_rpm] -> MTQD_LHMRollGenMapD_Z_Nm/2
  [VTQD_RollingShaftSpd_rpm] -> MTQD_LHMRollGenMapD_Z_Nm/1
  [VTQD_TqTargetShaftSpd_rpm] -> MTQD_LHMTqMapD_Z_Nm/2
  [VTQD_ActAPSPosn_pct] -> MTQD_LHMTqMapD_Z_Nm/1
  MTQD_LHMTqMapD_Z_Nm/1 -> [MTQD_LHMTqMapD_Z_Nm]
  VTQD_RollingShaftSpd_rpm/1 -> [VTQD_RollingShaftSpd_rpm]
  VTQD_RollRegenEnable_flg/1 -> [VTQD_RollRegenEnable_flg]
  VTQD_TqTargetShaftSpd_rpm/1 -> [VTQD_TqTargetShaftSpd_rpm]
  VTQD_ActAPSPosn_pct/1 -> [VTQD_ActAPSPosn_pct]

== system tqd/TQD/TorqueDemand/TorqueModule/DriverWhlTqDem/PedalMapWhlTq/LHM/ShiftPorN ==
  Action Port : ActionPort
  Constant : Constant  Value=ZERO_FLOAT
  VTQD_PedalMapWhlTqPorN_Nm : Outport
  wires:
  Constant/1 -> VTQD_PedalMapWhlTqPorN_Nm/1

== system tqd/TQD/TorqueDemand/TorqueModule/DriverWhlTqDem/PedalMapWhlTq/LHM/ShiftR ==
  VTQD_ActAPSPosn_pct : Inport
  VTQD_TqTargetShaftSpd_rpm : Inport  Port=2
  Action Port : ActionPort
  MTQD_LHMTqMapR_Z_Nm : Lookup_n-D  BreakpointsForDimension1=ATQD_LHMTqMapD_Y_pct  BreakpointsForDimension2=ATQD_LHMTqMapD_X_rpm  Table=MTQD_LHMTqMapR_Z_Nm  InternalRulePriority=Speed  RndMeth=Simplest  InputSameDT=on
      settings: InputPortMap=u0,u1
  VTQD_PedalMapWhlTqLHMR_Nm : Outport
  wires:
  [MTQD_LHMTqMapR_Z_Nm] -> VTQD_PedalMapWhlTqLHMR_Nm/1
  MTQD_LHMTqMapR_Z_Nm/1 -> [MTQD_LHMTqMapR_Z_Nm]
  [VTQD_ActAPSPosn_pct] -> MTQD_LHMTqMapR_Z_Nm/1
  [VTQD_TqTargetShaftSpd_rpm] -> MTQD_LHMTqMapR_Z_Nm/2
  VTQD_ActAPSPosn_pct/1 -> [VTQD_ActAPSPosn_pct]
  VTQD_TqTargetShaftSpd_rpm/1 -> [VTQD_TqTargetShaftSpd_rpm]

== system tqd/TQD/TorqueDemand/TorqueModule/DriverWhlTqDem/PedalMapWhlTq/NoLHM/ShiftD ==
  VTQD_EVDriveMode_enum : Inport
  VTQD_ActAPSPosn_pct : Inport  Port=2
  VTQD_TqTargetShaftSpd_rpm : Inport  Port=3
  VTQD_RegenMode_enum : Inport  Port=4
  VTQD_RollRegenEnable_flg : Inport  Port=5
  VTQD_RollingShaftSpd_rpm : Inport  Port=6
  VVMC_EstSlope_Deg : Inport  Port=7
  VTQD_APSReqTimer_s : Inport  Port=8
  VTQD_LowIdleAccPedal_flg : Inport  Port=9
  VTQD_OPDHoldEnRel_flg : Inport  Port=10
  VTQD_OPDHoldActRelTq_Nm : Inport  Port=11
  VTQD_VehActSpd_kph : Inport  Port=12
  VTQD_SlopeUp_flg : Inport  Port=13
  VINP_IVISnowModeCmd_flg : Inport  Port=14
  VTQD_PreDecTqLowLim_Nm : Inport  Port=15
  Action Port : ActionPort
  Constant5 : Constant  Value=ENUM_DRIVEMODE_NRM
  Constant6 : Constant  Value=ENUM_DRIVEMODE_ECO
  Constant7 : Constant  Value=ENUM_DRIVEMODE_SPORT
  Equal1 : RelationalOperator  Operator===  OutDataTypeStr=boolean  RndMeth=Simplest
  Equal2 : RelationalOperator  Operator===  OutDataTypeStr=boolean  RndMeth=Simplest
  Equal3 : RelationalOperator  Operator===  OutDataTypeStr=boolean  RndMeth=Simplest
  If : If  NumInputs=4  IfExpression=u1 ~= 0  ElseIfExpressions=u2 ~= 0,u3~=0
  LUT_D_ECO : Subsystem  TreatAsAtomicUnit=on
  LUT_D_Normal : Subsystem  TreatAsAtomicUnit=on
  LUT_D_SnowMode : Subsystem  TreatAsAtomicUnit=on
  LUT_D_Sport : Subsystem  TreatAsAtomicUnit=on
  Merge : Merge  Inputs=4
  VTQD_PedalMapWhlTqD_Nm : Outport
  wires:
  [VTQD_RollingShaftSpd_rpm] -> LUT_D_ECO/5(VTQD_RollingShaftSpd_rpm)
  [VTQD_RollRegenEnable_flg] -> LUT_D_ECO/4(VTQD_RollRegenEnable_flg)
  VTQD_RollingShaftSpd_rpm/1 -> [VTQD_RollingShaftSpd_rpm]
  VTQD_RollRegenEnable_flg/1 -> [VTQD_RollRegenEnable_flg]
  [VTQD_TqTargetShaftSpd_rpm] -> LUT_D_Sport/1(VTQD_TqTargetShaftSpd_rpm)
  [VTQD_ActAPSPosn_pct] -> LUT_D_Sport/2(VTQD_ActAPSPosn_pct)
  [VTQD_RegenMode_enum] -> LUT_D_Sport/3(VTQD_RegenMode_enum)
  [VTQD_RegenMode_enum] -> LUT_D_ECO/3(VTQD_RegenMode_enum)
  [VTQD_ActAPSPosn_pct] -> LUT_D_ECO/2(VTQD_ActAPSPosn_pct)
  [VTQD_TqTargetShaftSpd_rpm] -> LUT_D_ECO/1(VTQD_TqTargetShaftSpd_rpm)
  [VTQD_ActAPSPosn_pct] -> LUT_D_Normal/2(VTQD_ActAPSPosn_pct)
  [VTQD_TqTargetShaftSpd_rpm] -> LUT_D_Normal/1(VTQD_TqTargetShaftSpd_rpm)
  [VTQD_RegenMode_enum] -> LUT_D_Normal/3(VTQD_RegenMode_enum)
  VTQD_RegenMode_enum/1 -> [VTQD_RegenMode_enum]
  VTQD_TqTargetShaftSpd_rpm/1 -> [VTQD_TqTargetShaftSpd_rpm]
  VTQD_ActAPSPosn_pct/1 -> [VTQD_ActAPSPosn_pct]
  VTQD_EVDriveMode_enum/1 -> [VTQD_EVDriveMode_enum]
  Merge/1 -> VTQD_PedalMapWhlTqD_Nm/1
  Constant7/1 -> Equal3/2
  Constant5/1 -> Equal1/2
  [VTQD_EVDriveMode_enum] -> Equal3/1
  Constant6/1 -> Equal2/2
  [VTQD_EVDriveMode_enum] -> Equal2/1
  [VTQD_EVDriveMode_enum] -> Equal1/1
  [VVMC_EstSlope_Deg] -> LUT_D_Normal/4(VVMC_EstSlope_Deg)
  [VTQD_APSReqTimer_s] -> LUT_D_Normal/5(VTQD_APSReqTimer_s)
  VVMC_EstSlope_Deg/1 -> [VVMC_EstSlope_Deg]
  VTQD_APSReqTimer_s/1 -> [VTQD_APSReqTimer_s]
  [VVMC_EstSlope_Deg] -> LUT_D_ECO/6(VVMC_EstSlope_Deg)
  [VTQD_APSReqTimer_s] -> LUT_D_ECO/7(VTQD_APSReqTimer_s)
  [VVMC_EstSlope_Deg] -> LUT_D_Sport/4(VVMC_EstSlope_Deg)
  [VTQD_APSReqTimer_s] -> LUT_D_Sport/5(VTQD_APSReqTimer_s)
  [VTQD_LowIdleAccPedal_flg] -> LUT_D_Normal/6(VTQD_LowIdleAccPedal_flg)
  VTQD_LowIdleAccPedal_flg/1 -> [VTQD_LowIdleAccPedal_flg]
  [VTQD_LowIdleAccPedal_flg] -> LUT_D_ECO/8(VTQD_LowIdleAccPedal_flg)
  [VTQD_LowIdleAccPedal_flg] -> LUT_D_Sport/6(VTQD_LowIdleAccPedal_flg)
  VTQD_OPDHoldEnRel_flg/1 -> [VTQD_OPDHoldEnRel_flg]
  [VTQD_OPDHoldEnRel_flg] -> LUT_D_Normal/7(VTQD_OPDHoldEnRel_flg)
  VTQD_OPDHoldActRelTq_Nm/1 -> [VTQD_OPDHoldActRelTq_Nm]
  VTQD_VehActSpd_kph/1 -> [VTQD_VehActSpd_kph]
  [VTQD_VehActSpd_kph] -> LUT_D_Normal/9(VTQD_VehActSpd_kph)
  [VTQD_OPDHoldActRelTq_Nm] -> LUT_D_Normal/8(VTQD_OPDHoldActRelTq_Nm)
  [VTQD_OPDHoldEnRel_flg] -> LUT_D_ECO/9(VTQD_OPDHoldEnRel_flg)
  [VTQD_OPDHoldActRelTq_Nm] -> LUT_D_ECO/10(VTQD_OPDHoldActRelTq_Nm)
  [VTQD_VehActSpd_kph] -> LUT_D_ECO/11(VTQD_VehActSpd_kph)
  [VTQD_VehActSpd_kph] -> LUT_D_Sport/9(VTQD_VehActSpd_kph)
  [VTQD_OPDHoldActRelTq_Nm] -> LUT_D_Sport/8(VTQD_OPDHoldActRelTq_Nm)
  [VTQD_OPDHoldEnRel_flg] -> LUT_D_Sport/7(VTQD_OPDHoldEnRel_flg)
  VTQD_SlopeUp_flg/1 -> [VTQD_SlopeUp_flg]
  [VTQD_SlopeUp_flg] -> LUT_D_Normal/10(VTQD_SlopeUp_flg)
  [VTQD_SlopeUp_flg] -> LUT_D_Sport/10(VTQD_SlopeUp_flg)
  [VTQD_SlopeUp_flg] -> LUT_D_ECO/12(VTQD_SlopeUp_flg)
  If/2 -> LUT_D_Normal/Action
  If/3 -> LUT_D_ECO/Action
  If/4 -> LUT_D_Sport/Action
  Equal3/1 -> If/4
  Equal2/1 -> If/3
  Equal1/1 -> If/2
  [VINP_IVISnowModeCmd_flg] -> If/1
  [VTQD_TqTargetShaftSpd_rpm] -> LUT_D_SnowMode/1(VTQD_TqTargetShaftSpd_rpm)
  [VTQD_PreDecTqLowLim_Nm] -> LUT_D_SnowMode/4(VTQD_PreDecTqLowLim_Nm)
  [VTQD_ActAPSPosn_pct] -> LUT_D_SnowMode/2(VTQD_ActAPSPosn_pct)
  LUT_D_SnowMode/1(VTQD_WhlTqSnowMode_Nm) -> [VTQD_WhlTqSnowMode_Nm]  "VTQD_WhlTqSnowMode_Nm"
  If/1 -> LUT_D_SnowMode/Action
  [VTQD_RegenMode_enum] -> LUT_D_SnowMode/3(VTQD_RegenMode_enum)
  LUT_D_Normal/1(VTQD_WhlTqNRMD_Nm) -> [VTQD_WhlTqNRMD_Nm]  "VTQD_WhlTqNRMD_Nm"
  LUT_D_ECO/1(VTQD_WhlTqECOD_Nm) -> [VTQD_WhlTqECOD_Nm]  "VTQD_WhlTqECOD_Nm"
  LUT_D_Sport/1(VTQD_WhlTqSPORTD_Nm) -> [VTQD_WhlTqSPORTD_Nm]  "VTQD_WhlTqSPORTD_Nm"
  [VTQD_WhlTqSPORTD_Nm] -> Merge/4
  [VTQD_WhlTqSnowMode_Nm] -> Merge/1
  [VTQD_WhlTqECOD_Nm] -> Merge/3
  [VTQD_WhlTqNRMD_Nm] -> Merge/2
  VINP_IVISnowModeCmd_flg/1 -> [VINP_IVISnowModeCmd_flg]
  VTQD_PreDecTqLowLim_Nm/1 -> [VTQD_PreDecTqLowLim_Nm]

== system tqd/TQD/TorqueDemand/TorqueModule/DriverWhlTqDem/PedalMapWhlTq/NoLHM/ShiftPorN ==
  Action Port : ActionPort
  Constant : Constant  Value=ZERO_FLOAT
  VTQD_PedalMapWhlTqPorN_Nm : Outport
  wires:
  Constant/1 -> VTQD_PedalMapWhlTqPorN_Nm/1

== system tqd/TQD/TorqueDemand/TorqueModule/DriverWhlTqDem/PedalMapWhlTq/NoLHM/ShiftR ==
  VTQD_ActAPSPosn_pct : Inport
  VTQD_TqTargetShaftSpd_rpm : Inport  Port=2
  Action Port : ActionPort
  MTQD_NRMTqMapR_Z_Nm : Lookup_n-D  BreakpointsForDimension1=ATQD_NL1TqMapD_Y_pct  BreakpointsForDimension2=ATQD_NL1TqMapD_X_rpm  Table=MTQD_NRMTqMapR_Z_Nm  ExtrapMethod=Clip  InternalRulePriority=Speed  RndMeth=Simplest  InputSameDT=on
      settings: InputPortMap=u0,u1
  VTQD_PedalMapWhlTqR_Nm : Outport
  wires:
  [VTQD_NRMTqMapR_Nm] -> VTQD_PedalMapWhlTqR_Nm/1
  MTQD_NRMTqMapR_Z_Nm/1 -> [VTQD_NRMTqMapR_Nm]
  [VTQD_ActAPSPosn_pct] -> MTQD_NRMTqMapR_Z_Nm/1
  [VTQD_TqTargetShaftSpd_rpm] -> MTQD_NRMTqMapR_Z_Nm/2
  VTQD_ActAPSPosn_pct/1 -> [VTQD_ActAPSPosn_pct]
  VTQD_TqTargetShaftSpd_rpm/1 -> [VTQD_TqTargetShaftSpd_rpm]

== system tqd/TQD/TorqueDemand/TorqueModule/DriverWhlTqDem/PedalMapWhlTq/NoLHM/ShiftD/LUT_D_ECO ==
  VTQD_TqTargetShaftSpd_rpm : Inport
  VTQD_ActAPSPosn_pct : Inport  Port=2
  VTQD_RegenMode_enum : Inport  Port=3
  VTQD_RollRegenEnable_flg : Inport  Port=4
  VTQD_RollingShaftSpd_rpm : Inport  Port=5
  VVMC_EstSlope_Deg : Inport  Port=6
  VTQD_APSReqTimer_s : Inport  Port=7
  VTQD_LowIdleAccPedal_flg : Inport  Port=8
  VTQD_OPDHoldEnRel_flg : Inport  Port=9
  VTQD_OPDHoldActRelTq_Nm : Inport  Port=10
  VTQD_VehActSpd_kph : Inport  Port=11
  VTQD_SlopeUp_flg : Inport  Port=12
  Action Port : ActionPort  ActionPortLabel=elseif(u3~=0)
  Constant : Constant  Value=ENUM_REGENLEVEL_LV1
  Constant1 : Constant  Value=ENUM_REGENLEVEL_LV2
  Constant2 : Constant  Value=ENUM_REGENLEVEL_LV3
  Constant3 : Constant  Value=ENUM_REGENLEVEL_LV4
  Constant4 : Constant  Value=ENUM_REGENLEVEL_LV5
  Constant5 : Constant  Value=ENUM_REGENLEVEL_OPD
  ECO_Invalid_TqMap1 : Subsystem  TreatAsAtomicUnit=on
  ECO_Lv1_TqMap : Subsystem  TreatAsAtomicUnit=on
  ECO_Lv2_TqMap : Subsystem  TreatAsAtomicUnit=on
  ECO_Lv3_TqMap : Subsystem  TreatAsAtomicUnit=on
  ECO_Lv4_TqMap : Subsystem  TreatAsAtomicUnit=on
  ECO_Lv5_TqMap : Subsystem  TreatAsAtomicUnit=on
  ECO_OnePedal_TqMap : Subsystem  TreatAsAtomicUnit=on
  Equal{1..6} (6 alike) : RelationalOperator  Operator===  OutDataTypeStr=boolean  RndMeth=Simplest
  If : If  NumInputs=6  IfExpression=u1 ~= 0  ElseIfExpressions=u2 ~= 0, u3 ~= 0, u4 ~= 0, u5 ~= 0, u6 ~= 0
  MTQD_ECOTqMapD_Z_Nm : Lookup_n-D  BreakpointsForDimension1=ATQD_ECOTqMapD_Y_pct  BreakpointsForDimension2=ATQD_ECOTqMapD_X_rpm  Table=MTQD_ECOTqMapD_Z_Nm  ExtrapMethod=Clip  InternalRulePriority=Speed  RndMeth=Simplest  InputSameDT=on
      settings: InputPortMap=u0,u1
  MTQD_EL2TqMapD_Z_Nm : Lookup_n-D  BreakpointsForDimension1=ATQD_ECOTqMapD_Y_pct  BreakpointsForDimension2=ATQD_ECOTqMapD_X_rpm  Table=MTQD_EL2TqMapD_Z_Nm  ExtrapMethod=Clip  InternalRulePriority=Speed  RndMeth=Simplest  InputSameDT=on
      settings: InputPortMap=u0,u1
  MTQD_EL3TqMapD_Z_Nm : Lookup_n-D  BreakpointsForDimension1=ATQD_ECOTqMapD_Y_pct  BreakpointsForDimension2=ATQD_ECOTqMapD_X_rpm  Table=MTQD_EL3TqMapD_Z_Nm  ExtrapMethod=Clip  InternalRulePriority=Speed  RndMeth=Simplest  InputSameDT=on
      settings: InputPortMap=u0,u1
  MTQD_EL4TqMapD_Z_Nm : Lookup_n-D  BreakpointsForDimension1=ATQD_ECOTqMapD_Y_pct  BreakpointsForDimension2=ATQD_ECOTqMapD_X_rpm  Table=MTQD_EL4TqMapD_Z_Nm  ExtrapMethod=Clip  InternalRulePriority=Speed  RndMeth=Simplest  InputSameDT=on
      settings: InputPortMap=u0,u1
  MTQD_EL5TqMapD_Z_Nm : Lookup_n-D  BreakpointsForDimension1=ATQD_ECOTqMapD_Y_pct  BreakpointsForDimension2=ATQD_ECOTqMapD_X_rpm  Table=MTQD_EL5TqMapD_Z_Nm  ExtrapMethod=Clip  InternalRulePriority=Speed  RndMeth=Simplest  InputSameDT=on
      settings: InputPortMap=u0,u1
  MTQD_EOPDTqMapDCon_Z_Nm : Lookup_n-D  BreakpointsForDimension1=ATQD_EOPDTqMapDCon_Y_Deg  BreakpointsForDimension2=ATQD_EOPDTqMapDCon_X_rpm  Table=MTQD_EOPDTqMapDCon_Z_Nm  ExtrapMethod=Clip  InternalRulePriority=Speed  RndMeth=Simplest  InputSameDT=on
      settings: InputPortMap=u0,u1
  MTQD_EOPDTqMapD_Z_Nm : Lookup_n-D  BreakpointsForDimension1=ATQD_ECOTqMapD_Y_pct  BreakpointsForDimension2=ATQD_ECOTqMapD_X_rpm  Table=MTQD_EOPDTqMapD_Z_Nm  ExtrapMethod=Clip  InternalRulePriority=Speed  RndMeth=Simplest  InputSameDT=on
      settings: InputPortMap=u0,u1
  MTQD_RollGenMapEL1_Z_Nm : Lookup_n-D  BreakpointsForDimension1=ATQD_RollGenMapEL1_Y_rpm  BreakpointsForDimension2=ATQD_RollGenMapEL1_X_rpm  Table=MTQD_RollGenMapEL1_Z_Nm  ExtrapMethod=Clip  InternalRulePriority=Speed  RndMeth=Simplest  InputSameDT=on
      settings: InputPortMap=u0,u1
  Merge : Merge  Inputs=7
  VTQD_WhlTqECOD_Nm : Outport
  wires:
  [VTQD_ECOTqMapD_Nm] -> ECO_Lv1_TqMap/3(MTQD_ECOTqMapD_Z_Nm)
  [VTQD_RollGenMapEL1_Nm] -> ECO_Lv1_TqMap/2(MTQD_RollGenMapEL1_Z_Nm)
  [VTQD_RollRegenEnable_flg] -> ECO_Lv1_TqMap/1(VTQD_RollRegenEnable_flg)
  [VTQD_TqTargetShaftSpd_rpm] -> MTQD_RollGenMapEL1_Z_Nm/2
  [VTQD_RollingShaftSpd_rpm] -> MTQD_RollGenMapEL1_Z_Nm/1
  MTQD_RollGenMapEL1_Z_Nm/1 -> [VTQD_RollGenMapEL1_Nm]
  VTQD_RollingShaftSpd_rpm/1 -> [VTQD_RollingShaftSpd_rpm]
  VTQD_RollRegenEnable_flg/1 -> [VTQD_RollRegenEnable_flg]
  Equal6/1 -> If/6
  [VTQD_RegenMode_enum] -> Equal6/1
  Constant5/1 -> Equal6/2
  Equal5/1 -> If/5
  [VTQD_RegenMode_enum] -> Equal5/1
  Constant4/1 -> Equal5/2
  Equal4/1 -> If/4
  [VTQD_RegenMode_enum] -> Equal4/1
  Constant3/1 -> Equal4/2
  [VTQD_RegenMode_enum] -> Equal3/1
  Constant2/1 -> Equal3/2
  [VTQD_RegenMode_enum] -> Equal2/1
  Constant1/1 -> Equal2/2
  Constant/1 -> Equal1/2
  [VTQD_RegenMode_enum] -> Equal1/1
  [VTQD_EOPDTqMapD_Nm] -> ECO_OnePedal_TqMap/1(VTQD_EOPDTqMapDIn_Nm)
  If/6 -> ECO_OnePedal_TqMap/Action
  ECO_OnePedal_TqMap/1(VTQD_EOPDTqMapDOut_Nm) -> Merge/6
  [VTQD_EL5TqMapD_Nm] -> ECO_Lv5_TqMap/1(VTQD_EL5TqMapDIn_Nm)
  If/5 -> ECO_Lv5_TqMap/Action
  ECO_Lv5_TqMap/1(VTQD_EL5TqMapDOut_Nm) -> Merge/5
  ECO_Lv4_TqMap/1(VTQD_EL4TqMapDOut_Nm) -> Merge/4
  If/4 -> ECO_Lv4_TqMap/Action
  [VTQD_EL4TqMapD_Nm] -> ECO_Lv4_TqMap/1(VTQD_EL4TqMapDIn_Nm)
  [VTQD_EL3TqMapD_Nm] -> ECO_Lv3_TqMap/1(VTQD_EL3TqMapDIn_Nm)
  If/3 -> ECO_Lv3_TqMap/Action
  ECO_Lv3_TqMap/1(VTQD_EL3TqMapDOut_Nm) -> Merge/3
  [VTQD_EL2TqMapD_Nm] -> ECO_Lv2_TqMap/1(VTQD_EL2TqMapDIn_Nm)
  ECO_Lv2_TqMap/1(VTQD_EL2TqMapDOut_Nm) -> Merge/2
  If/2 -> ECO_Lv2_TqMap/Action
  ECO_Lv1_TqMap/1(VTQD_EL1TqMapDOut_Nm) -> Merge/1
  Equal1/1 -> If/1
  Equal2/1 -> If/2
  If/1 -> ECO_Lv1_TqMap/Action
  Merge/1 -> VTQD_WhlTqECOD_Nm/1
  Equal3/1 -> If/3
  [VTQD_TqTargetShaftSpd_rpm] -> MTQD_EOPDTqMapD_Z_Nm/2
  [VTQD_ActAPSPosn_pct] -> MTQD_EOPDTqMapD_Z_Nm/1
  [VTQD_TqTargetShaftSpd_rpm] -> MTQD_EL5TqMapD_Z_Nm/2
  [VTQD_ActAPSPosn_pct] -> MTQD_EL5TqMapD_Z_Nm/1
  [VTQD_TqTargetShaftSpd_rpm] -> MTQD_EL3TqMapD_Z_Nm/2
  [VTQD_ActAPSPosn_pct] -> MTQD_EL3TqMapD_Z_Nm/1
  [VTQD_TqTargetShaftSpd_rpm] -> MTQD_EL2TqMapD_Z_Nm/2
  [VTQD_ActAPSPosn_pct] -> MTQD_EL2TqMapD_Z_Nm/1
  MTQD_EL5TqMapD_Z_Nm/1 -> [VTQD_EL5TqMapD_Nm]
  MTQD_EL4TqMapD_Z_Nm/1 -> [VTQD_EL4TqMapD_Nm]
  [VTQD_TqTargetShaftSpd_rpm] -> MTQD_EL4TqMapD_Z_Nm/2
  [VTQD_ActAPSPosn_pct] -> MTQD_EL4TqMapD_Z_Nm/1
  MTQD_EOPDTqMapD_Z_Nm/1 -> [VTQD_EOPDTqMapD_Nm]
  MTQD_EL3TqMapD_Z_Nm/1 -> [VTQD_EL3TqMapD_Nm]
  MTQD_EL2TqMapD_Z_Nm/1 -> [VTQD_EL2TqMapD_Nm]
  [VTQD_ActAPSPosn_pct] -> MTQD_ECOTqMapD_Z_Nm/1
  [VTQD_TqTargetShaftSpd_rpm] -> MTQD_ECOTqMapD_Z_Nm/2
  VTQD_RegenMode_enum/1 -> [VTQD_RegenMode_enum]
  VTQD_ActAPSPosn_pct/1 -> [VTQD_ActAPSPosn_pct]
  VTQD_TqTargetShaftSpd_rpm/1 -> [VTQD_TqTargetShaftSpd_rpm]
  MTQD_ECOTqMapD_Z_Nm/1 -> [VTQD_ECOTqMapD_Nm]
  ECO_Invalid_TqMap1/1(VTQD_EL1TqMapDOut_Nm) -> Merge/7
  [VTQD_RollRegenEnable_flg] -> ECO_Invalid_TqMap1/1(VTQD_RollRegenEnable_flg)
  [VTQD_RollGenMapEL1_Nm] -> ECO_Invalid_TqMap1/2(MTQD_RollGenMapEL1_Z_Nm)
  [VTQD_ECOTqMapD_Nm] -> ECO_Invalid_TqMap1/3(MTQD_ECOTqMapD_Z_Nm)
  If/7 -> ECO_Invalid_TqMap1/Action
  [VTQD_TqTargetShaftSpd_rpm] -> MTQD_EOPDTqMapDCon_Z_Nm/2
  [VVMC_EstSlope_Deg] -> MTQD_EOPDTqMapDCon_Z_Nm/1
  MTQD_EOPDTqMapDCon_Z_Nm/1 -> [VTQD_EOPDTqMapDCon_Nm]
  VVMC_EstSlope_Deg/1 -> [VVMC_EstSlope_Deg]
  VTQD_APSReqTimer_s/1 -> [VTQD_APSReqTimer_s]
  [VTQD_EOPDTqMapDCon_Nm] -> ECO_OnePedal_TqMap/2(VTQD_EOPDTqMapDCon_Nm)
  [VTQD_APSReqTimer_s] -> ECO_OnePedal_TqMap/3(VTQD_APSReqTimer_s)
  [VTQD_LowIdleAccPedal_flg] -> ECO_OnePedal_TqMap/4(VTQD_LowIdleAccPedal_flg)
  VTQD_LowIdleAccPedal_flg/1 -> [VTQD_LowIdleAccPedal_flg]
  VTQD_OPDHoldActRelTq_Nm/1 -> [VTQD_OPDHoldActRelTq_Nm]
  VTQD_OPDHoldEnRel_flg/1 -> [VTQD_OPDHoldEnRel_flg]
  VTQD_VehActSpd_kph/1 -> [VTQD_VehActSpd_kph]
  [VTQD_VehActSpd_kph] -> ECO_OnePedal_TqMap/7(VTQD_VehActSpd_kph)
  [VTQD_OPDHoldActRelTq_Nm] -> ECO_OnePedal_TqMap/6(VTQD_OPDHoldActRelTq_Nm)
  [VTQD_OPDHoldEnRel_flg] -> ECO_OnePedal_TqMap/5(VTQD_OPDHoldEnRel_flg)
  VTQD_SlopeUp_flg/1 -> [VTQD_SlopeUp_flg]
  [VTQD_SlopeUp_flg] -> ECO_OnePedal_TqMap/8(VTQD_SlopeUp_flg)
